simulink model "encoder_test"  (R2022b)
settings: Solver=FixedStepDiscrete  StartTime=0.0  StopTime=10.0  FixedStep=1/500000  RelTol=1e-3
undefined symbols (not defined in the file or in its folder): ee_sli_rtmsupport, gcbh
libraries: simulink x4, spsSawtoothGeneratorLib x1
settings Model: Creator=dwegg  LastModifiedBy=dwegg

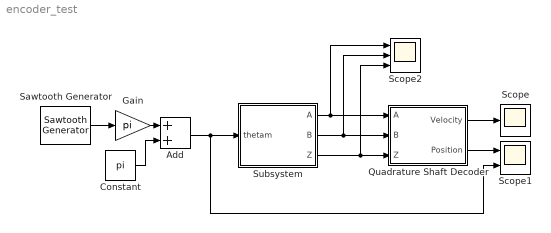
== system encoder_test ==
  Add : Sum
  Constant : Constant  Value=pi
  Gain : Gain  Gain=pi
  Quadrature Shaft Decoder : Subsystem  AncestorBlock=ee_sl_lib/Observers/Quadrature Shaft Decoder  LoadFcn=ee_sli_rtmsupport( 'loadfcn', gcbh );  mask(Quadrature Shaft Decoder){NPulse=4096, Ts=1/50000}
      mask prompts: NPulse "physmod:ee:library:comments:control:eeQuadratureDecoder:PulsesPerRevolutio_MP"; Ts "physmod:ee:library:comments:control:eeQuadratureDecoder:SampleTime1ForInherited_MP"
      mask help: physmod:ee:library:comments:control:eeQuadratureDecoder:QuadratureDecoder_MD
      mask init:
      | if Ts <= 0 && Ts ~= -1            
      |     error(message('physmod:ee:library:MinusOneOrPositive',getString(message('physmod:ee:library:comments:control:eeResolverToDigitalConverter:SampleTime1ForInherited_MP'))));            
      | end
      | 
      | if NPulse <= 0          
      |     error(message('physmod:simscape:compiler:patterns:checks:GreaterThanZero',getString(message('physmod:ee:library:comments:control:eeQuadratureDecoder:PulsesPerRevolutio_MP'))));            
      | end
      settings: CopyFcn=ee_sli_rtmsupport( 'copyfcn', gcbh );  DeleteFcn=ee_sli_rtmsupport( 'deletefcn', gcbh );  ModelCloseFcn=ee_sli_rtmsupport( 'modelclosefcn', gcbh );  PostSaveFcn=ee_sli_rtmsupport( 'postsavefcn', gcbh );  PreCopyFcn=ee_sli_rtmsupport( 'precopyfcn', gcbh );  OpenFcn=ee_sli_rtmsupport( 'openfcn', gcbh );  CloseFcn=ee_sli_rtmsupport( 'closefcn', gcbh );  PreDeleteFcn=ee_sli_rtmsupport( 'predeletefcn', gcbh );
      settings: LibrarySourceBlock=|
      | ee_sl_lib/Observers/Quadrature Shaft
      | Decoder
      mask Help: web(nesl_help(gcbh))
      mask DialogControl NPulse Prompt: Pulses per revolution
      mask DialogControl Ts Prompt: Sample time (-1 for inherited)
  Sawtooth Generator : spsSawtoothGeneratorLib/Sawtooth Generator  Freq=1e2  Phase=180  Ts=0
  Scope : Scope
  Scope1 : Scope  NumInputPorts=2
  Scope2 : Scope  NumInputPorts=3
  Subsystem : Subsystem
  wires:
  Subsystem/1(A) -> Scope2/1, Quadrature Shaft Decoder/1(A)
  Subsystem/2(B) -> Scope2/2, Quadrature Shaft Decoder/2(B)
  Subsystem/3(Z) -> Scope2/3, Quadrature Shaft Decoder/3(Z)
  Sawtooth Generator/1 -> Gain/1
  Quadrature Shaft Decoder/1(Velocity) -> Scope/1
  Quadrature Shaft Decoder/2(Position) -> Scope1/1
  Add/1 -> Subsystem/1(thetam), Scope1/2
  Gain/1 -> Add/1
  Constant/1 -> Add/2

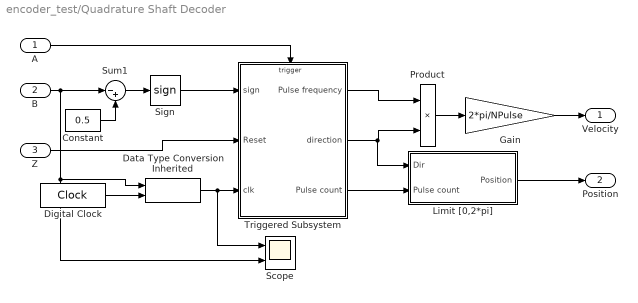
== system encoder_test/Quadrature Shaft Decoder ==
  A : Inport  SampleTime=Ts
  B : Inport  Port=2  SampleTime=Ts
  Z : Inport  Port=3  SampleTime=Ts
  Constant : Constant  Value=0.5  SampleTime=Ts
  Data Type Conversion Inherited : simulink/Signal Attributes/Data Type Conversion Inherited  ConvertRealWorld=Real World Value  DoSatur=off
  Digital Clock : DigitalClock  SampleTime=Ts
  Gain : Gain  Gain=2*pi/NPulse
  Limit [0,2*pi] : Subsystem
  Product : Product
  Scope : Scope  NumInputPorts=2
  Sign : Signum
  Sum1 : Sum  Inputs=|-+  OutDataTypeStr=Inherit: Same as first input
  Triggered Subsystem : Subsystem  TreatAsAtomicUnit=on
  Velocity : Outport  VectorParamsAs1DForOutWhenUnconnected=off
  Position : Outport  Port=2  VectorParamsAs1DForOutWhenUnconnected=off
  wires:
  Sign/1 -> Triggered Subsystem/1(sign)
  A/1 -> Triggered Subsystem/Trigger
  B/1 -> Scope/2, Data Type Conversion Inherited/1, Sum1/1
  Sum1/1 -> Sign/1
  Constant/1 -> Sum1/2
  Triggered Subsystem/1(Pulse frequency) -> Product/1
  Triggered Subsystem/2(direction) -> Limit [0,2*pi]/1(Dir), Product/2
  Product/1 -> Gain/1
  Gain/1 -> Velocity/1
  Z/1 -> Triggered Subsystem/2(Reset)
  Triggered Subsystem/3(Pulse count) -> Limit [0,2*pi]/2(Pulse count)
  Limit [0,2*pi]/1(Position) -> Position/1
  Data Type Conversion Inherited/1 -> Scope/1, Triggered Subsystem/3(clk)
  Digital Clock/1 -> Data Type Conversion Inherited/2

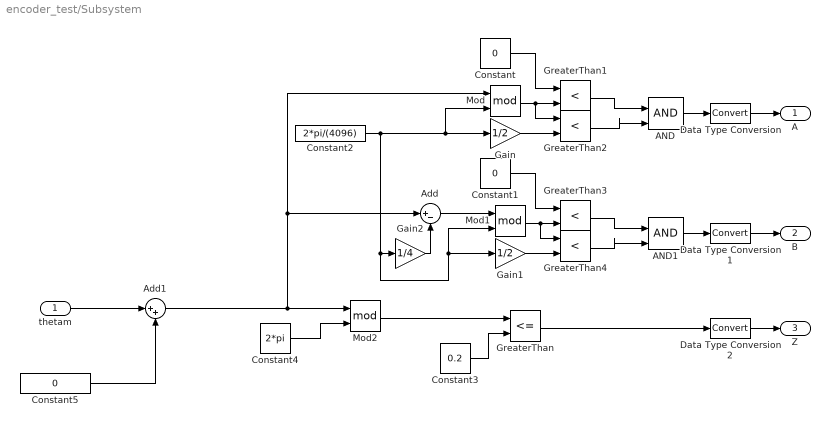
== system encoder_test/Subsystem ==
  thetam : Inport
  AND : Logic  IconShape=distinctive  AllPortsSameDT=off  OutDataTypeStr=boolean
  AND1 : Logic  IconShape=distinctive  AllPortsSameDT=off  OutDataTypeStr=boolean
  Add : Sum  Inputs=|+-
  Add1 : Sum  Inputs=|++
  Constant : Constant  Value=0
  Constant1 : Constant  Value=0
  Constant2 : Constant  Value=2*pi/(4096)
  Constant3 : Constant  Value=0.2
  Constant4 : Constant  Value=2*pi
  Constant5 : Constant  Value=0
  Data Type Conversion : DataTypeConversion  SaturateOnIntegerOverflow=off  RndMeth=Floor
  Data Type Conversion1 : DataTypeConversion  SaturateOnIntegerOverflow=off  RndMeth=Floor
  Data Type Conversion2 : DataTypeConversion  SaturateOnIntegerOverflow=off  RndMeth=Floor
  Gain : Gain  Gain=1/2
  Gain1 : Gain  Gain=1/2
  Gain2 : Gain  Gain=1/4
  GreaterThan : RelationalOperator  Operator=<=  OutDataTypeStr=boolean  RndMeth=Simplest  InputSameDT=off
  GreaterThan{1..4} (4 alike) : RelationalOperator  Operator=<  OutDataTypeStr=boolean  RndMeth=Simplest  InputSameDT=off
  Mod : Math  Operator=mod
  Mod1 : Math  Operator=mod
  Mod2 : Math  Operator=mod
  A : Outport
  B : Outport  Port=2
  Z : Outport  Port=3
  wires:
  AND/1 -> Data Type Conversion/1
  AND1/1 -> Data Type Conversion1/1
  GreaterThan1/1 -> AND/1
  GreaterThan2/1 -> AND/2
  GreaterThan4/1 -> AND1/2
  GreaterThan3/1 -> AND1/1
  Constant/1 -> GreaterThan1/1
  Constant1/1 -> GreaterThan3/1
  Mod/1 -> GreaterThan2/1, GreaterThan1/2
  Gain/1 -> GreaterThan2/2
  Add1/1 -> Add/1, Mod/1, Mod2/1
  Constant2/1 -> Mod/2, Gain/1, Gain2/1, Gain1/1, Mod1/2
  Mod1/1 -> GreaterThan4/1, GreaterThan3/2
  Gain1/1 -> GreaterThan4/2
  Add/1 -> Mod1/1
  Gain2/1 -> Add/2
  GreaterThan/1 -> Data Type Conversion2/1
  Constant3/1 -> GreaterThan/2
  Mod2/1 -> GreaterThan/1
  Constant4/1 -> Mod2/2
  thetam/1 -> Add1/1
  Constant5/1 -> Add1/2
  Data Type Conversion/1 -> A/1
  Data Type Conversion1/1 -> B/1
  Data Type Conversion2/1 -> Z/1

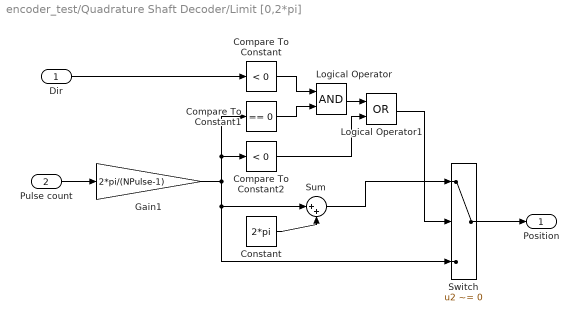
== system encoder_test/Quadrature Shaft Decoder/Limit [0,2*pi] ==
  Dir : Inport
  Pulse count : Inport  Port=2
  Compare To Constant : simulink/Logic and Bit Operations/Compare To Constant  relop=<  const=0  OutDataTypeStr=boolean
  Compare To Constant1 : simulink/Logic and Bit Operations/Compare To Constant  relop===  const=0  OutDataTypeStr=boolean
  Compare To Constant2 : simulink/Logic and Bit Operations/Compare To Constant  relop=<  const=0  OutDataTypeStr=boolean
  Constant : Constant  Value=2*pi
  Gain1 : Gain  Gain=2*pi/(NPulse-1)
  Logical Operator : Logic  AllPortsSameDT=off  OutDataTypeStr=boolean
  Logical Operator1 : Logic  Operator=OR  AllPortsSameDT=off  OutDataTypeStr=boolean
  Sum : Sum  Inputs=|++  OutDataTypeStr=Inherit: Same as first input
  Switch : Switch  Criteria=u2 ~= 0  SaturateOnIntegerOverflow=off  InputSameDT=off
  Position : Outport  VectorParamsAs1DForOutWhenUnconnected=off
  wires:
  Pulse count/1 -> Gain1/1
  Dir/1 -> Compare To Constant/1
  Sum/1 -> Switch/1
  Compare To Constant/1 -> Logical Operator/1
  Compare To Constant1/1 -> Logical Operator/2
  Logical Operator/1 -> Logical Operator1/1
  Switch/1 -> Position/1
  Compare To Constant2/1 -> Logical Operator1/2
  Logical Operator1/1 -> Switch/2
  Gain1/1 -> Sum/1, Switch/3, Compare To Constant2/1, Compare To Constant1/1
  Constant/1 -> Sum/2

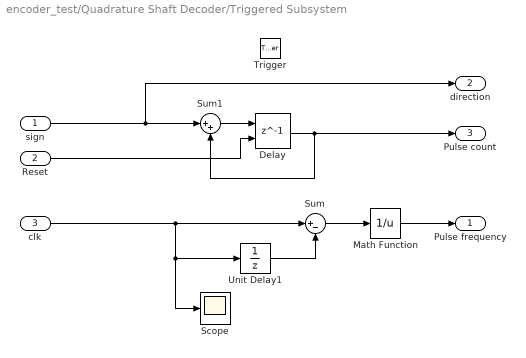
== system encoder_test/Quadrature Shaft Decoder/Triggered Subsystem ==
  sign : Inport
  Reset : Inport  Port=2
  clk : Inport  Port=3
  Trigger : TriggerPort  VariantControl=Variant
  Delay : Delay  DelayLength=1  InitialCondition=0  ExternalReset=Rising
      settings: InputPortMap=u0,r5
  Math Function : Math  Operator=reciprocal  SignedPower=on
  Scope : Scope
  Sum : Sum  Inputs=|+-  OutDataTypeStr=Inherit: Same as first input
  Sum1 : Sum  Inputs=|++  OutDataTypeStr=Inherit: Same as first input
  Unit Delay1 : UnitDelay  InitialCondition=-1e10  SampleTime=-1  HasFrameUpgradeWarning=on
  Pulse frequency : Outport  VectorParamsAs1DForOutWhenUnconnected=off
  direction : Outport  Port=2  InitialOutput=0  VectorParamsAs1DForOutWhenUnconnected=off
  Pulse count : Outport  Port=3  InitialOutput=0  VectorParamsAs1DForOutWhenUnconnected=off
  wires:
  Sum1/1 -> Delay/1
  sign/1 -> Sum1/1, direction/1
  Delay/1 -> Pulse count/1, Sum1/2
  clk/1 -> Scope/1, Unit Delay1/1, Sum/1
  Unit Delay1/1 -> Sum/2
  Sum/1 -> Math Function/1
  Math Function/1 -> Pulse frequency/1
  Reset/1 -> Delay/2
